simulink model "EKF"  (R2021b)
settings: Solver=ode4  StartTime=0.0  StopTime=200  FixedStep=0.02  RelTol=1e-3
libraries: commchan3 x2
(part 2 of 4)

== matlab function EKF/MATLAB Function3 ==
  data: y input; xhat output; u input; Pcov output; xhat input
function [xhat, Pcov]= fcn(y, u, xhat)
    Ts = 0.02;
    Qk = eye(5);
    Qk(1,1) = 1e-8;
    Qk(2,2) = 1e-8;
    Qk(3,3) = 1e-8;
    Qk(4,4) = 1e-5;
    Qk(5,5) = 1e-2;
    Rk = 1e-6;
    C = [0, 1, 0, 0, 0];
    n = 5; % dimension of state space
    lambda=(alpha)^2+(n+k)-n;
    alpha=1e-3;
    beta = 2;
    k=0;

   
    W_0m=lambda/(n+lambda);
    W_0c=W_mo+(1-(alpha)^2+beta);

%     for i = 1:2*n
        W_0m1 = 1/(2*(n+lambda));
%     end
    
   
    persistent xhat_p mhat_p Pcov_p xhata_p phata_p;

    % initialization
    if isempty(xhat_p)
        xhat_p = [0;0;0;1/2;4];
        Pcov_p = (xhat_p - mhat_p)* (xhat_p - mhat_p)';
    end

    W_0m=lambda/(n+lambda);
    x_sigma0 = xhat_p;
    x_sigma1 = zeros(5,1);
    x_sigma2 = zeros(5,1);
%     x_sigma = zeros(10,1);

    for i=1:n
        x_sigma1(i) = xhat_p+sqrt((n+lambda)*Pcov_p(i));
    end

    for i=n+1:2*n
        x_sigma2(i) = xhat_p-sqrt((n+lambda)*Pcov_p(i));
    end
    

%    xkm = Fd(x_sigma, u, Ts);
    x_prior=zeros(5,1);
    x_prior1=zeros(5,1);
    x_prior2=zeros(5,1);
    x_prior3=zeros(5,1);
    P_prior=zeros(5,5);
    P_prior1=zeros(5,5);
    P_prior2=zeros(5,5);
    P_prior3=zeros(5,5);
    y_prior=zeros(5,1);

    for i = 1:(2*n+1)
        if i == 1
            x_prior1 = x_prior + W_0m * x_sigma0;
        elseif i > 1 && i <= n
            x_prior2(i) =  x_prior2(i) + W_0m1 *x_sigma1(i);
        elseif i > n && i <= (2*n+1)
             x_prior3(i) =  x_prior3(i) + W_0m1 *x_sigma2(i);
        end
    end

    x_prior = x_prior1 + x_prior2 + x_prior3;

   for i = 1:(2*n+1)
        if i == 1
            P_prior1 = P_prior1 + W_0c * [x_sigma0 - x_prior] * [x_sigma0 - x_prior]';
        elseif i > 1 && i <= n
            P_prior2(i) = P_prior2(i) + W_0m1   * [x_sigma1(i) - x_prior] * [x_sigma1(i) - x_prior]';
        elseif i > n && i <= (2*n+1)
            P_prior3(i) = P_prior3(i) + W_0m1   * [x_sigma3(i) - x_prior] * [x_sigma3(i) - x_prior]';
        end
   end

   P_prior = P_prior1 + P_prior2 + P_prior3;

 y_sigma0 = y;
    y_sigma1 = zeros(5,1);
    y_sigma2 = zeros(5,1);


    for i=1:n
        y_sigma1(i) = y+sqrt((n+lambda)*Pcov_p(i));
    end

    for i=n+1:2*n
        y_sigma2(i) = y-sqrt((n+lambda)*Pcov_p(i));
    end

     y_prior=zeros(5,1);
    y_prior1=zeros(5,1);
    y_prior2=zeros(5,1);
    y_prior3=zeros(5,1);
for i = 1:(2*n+1)
        if i == 1
            y_prior1 = y_prior + W_0m1 * y_sigma0;
        elseif i > 1 && i <= n
            y_prior2(i) =  y_prior2(i) + W_0m1 *y_sigma1(i);
        elseif i > n && i <= (2*n+1)
             y_prior3(i) =  y_prior3(i) + W_0m1 *y_sigma2(i);
        end
    end
end
    y_prior = y_prior1 + y_prior2 + y_prior3;

    %measurement update
    Pyy=zeros(5,5);
    Pxy=zeros(5,5);

   
   for i = 1:(2*n+1)
        if i == 1
            P_prior1 = P_prior1 + W_0c * [y_sigma0 - y_prior] * [x_sigma0 - x_prior]';
        elseif i > 1 && i <= n
            P_prior2(i) = P_prior2(i) + W_0m1   * [x_sigma1(i) - x_prior] * [x_sigma1(i) - x_prior]';
        elseif i > n && i <= (2*n+1)
            P_prior3(i) = P_prior3(i) + W_0m1   * [x_sigma3(i) - x_prior] * [x_sigma3(i) - x_prior]';
        end
   end

   P_prior = P_prior1 + P_prior2 + P_prior3

%     
%     Fk = J_wrtX(xhat_p, u, Ts);
%     Pkm = Fk*Pcov_p*Fk' + Qk;
%     
%     y_err = y - C*xkm;
%     Sk = C*Pkm*C' + Rk;
%     Kk = Pkm * C'*inv(Sk);
%     xhat = xkm + Kk*y_err;
%     Pcov_final = (eye(5) - Kk*C)*Pkm;
%     
%     Pcov = reshape(Pcov_final, [25, 1]);
%     
%     xhat_p = xhat;
%     Pcov_p = Pcov_final;
% 
%     function X1 = Fd(x, u, Ts)
%         x1 = x(1);
%         x2 = x(2);
%         x3 = x(3);
%         M = x(4);
%         D = x(5);
%         X1 = [x1 + (Ts*(6*x2 + Ts*x3 + Ts*(x3 - (Ts*(5*M*u + (x2 + (Ts*x3)/2)*(100*M + 5*D*M) + 10*M*(x1 + (Ts*x2)/2) + (x3 - (Ts*(5*M*u + 10*M*x1 + x3*(D*M + 5) + x2*(100*M + 5*D*M)))/2)*(D*M + 5)))/2) + Ts*(x3 - (Ts*(5*M*u + 10*M*x1 + x3*(D*M + 5) + x2*(100*M + 5*D*M)))/2)))/6;
%              x2 - (Ts*(Ts*(5*M*u + (x2 + (Ts*x3)/2)*(100*M + 5*D*M) + 10*M*(x1 + (Ts*x2)/2) + (x3 - (Ts*(5*M*u + 10*M*x1 + x3*(D*M + 5) + x2*(100*M + 5*D*M)))/2)*(D*M + 5)) - 6*x3 + Ts*((x2 + (Ts*(x3 - (Ts*(5*M*u + 10*M*x1 + x3*(D*M + 5) + x2*(100*M + 5*D*M)))/2))/2)*(100*M + 5*D*M) + 5*M*u + 10*M*(x1 + (Ts*(x2 + (Ts*x3)/2))/2) + (D*M + 5)*(x3 - (Ts*(5*M*u + (x2 + (Ts*x3)/2)*(100*M + 5*D*M) + 10*M*(x1 + (Ts*x2)/2) + (x3 - (Ts*(5*M*u + 10*M*x1 + x3*(D*M + 5) + x2*(100*M + 5*D*M)))/2)*(D*M + 5)))/2)) + Ts*(5*M*u + 10*M*x1 + x3*(D*M + 5) + x2*(100*M + 5*D*M))))/6;
%              x3 - (Ts*(2*(x2 + (Ts*(x3 - (Ts*(5*M*u + 10*M*x1 + x3*(D*M + 5) + x2*(100*M + 5*D*M)))/2))/2)*(100*M + 5*D*M) + 30*M*u + 10*M*x1 + x3*(D*M + 5) + 20*M*(x1 + (Ts*(x2 + (Ts*x3)/2))/2) + 2*(x2 + (Ts*x3)/2)*(100*M + 5*D*M) + 2*(D*M + 5)*(x3 - (Ts*(5*M*u + (x2 + (Ts*x3)/2)*(100*M + 5*D*M) + 10*M*(x1 + (Ts*x2)/2) + (x3 - (Ts*(5*M*u + 10*M*x1 + x3*(D*M + 5) + x2*(100*M + 5*D*M)))/2)*(D*M + 5)))/2) + 20*M*(x1 + (Ts*x2)/2) + (x3 - Ts*((x2 + (Ts*(x3 - (Ts*(5*M*u + 10*M*x1 + x3*(D*M + 5) + x2*(100*M + 5*D*M)))/2))/2)*(100*M + 5*D*M) + 5*M*u + 10*M*(x1 + (Ts*(x2 + (Ts*x3)/2))/2) + (D*M + 5)*(x3 - (Ts*(5*M*u + (x2 + (Ts*x3)/2)*(100*M + 5*D*M) + 10*M*(x1 + (Ts*x2)/2) + (x3 - (Ts*(5*M*u + 10*M*x1 + x3*(D*M + 5) + x2*(100*M + 5*D*M)))/2)*(D*M + 5)))/2)))*(D*M + 5) + x2*(100*M + 5*D*M) + 2*(x3 - (Ts*(5*M*u + 10*M*x1 + x3*(D*M + 5) + x2*(100*M + 5*D*M)))/2)*(D*M + 5) + (x2 + Ts*(x3 - (Ts*(5*M*u + (x2 + (Ts*x3)/2)*(100*M + 5*D*M) + 10*M*(x1 + (Ts*x2)/2) + (x3 - (Ts*(5*M*u + 10*M*x1 + x3*(D*M + 5) + x2*(100*M + 5*D*M)))/2)*(D*M + 5)))/2))*(100*M + 5*D*M) + 10*M*(x1 + Ts*(x2 + (Ts*(x3 - (Ts*(5*M*u + 10*M*x1 + x3*(D*M + 5) + x2*(100*M + 5*D*M)))/2))/2))))/6;
%              M;
%              D];
%     end
% 
%     function Ad = J_wrtX(x, u, Ts)
%         x1 = x(1);
%         x2 = x(2);
%         x3 = x(3);
%         M = x(4);
%         D = x(5);
%         Ad = [1 - (Ts*(5*M*Ts^2 + (Ts^2*(10*M - 5*M*Ts*(D*M + 5)))/2))/6,-(Ts*((Ts^2*(100*M + 5*D*M))/2 + (Ts^2*(100*M + 5*M*Ts + 5*D*M - (Ts*(D*M + 5)*(100*M + 5*D*M))/2))/2 - 6))/6, (Ts*(Ts - Ts*((Ts*(D*M + 5))/2 - 1) + Ts*((Ts*((D*M + 5)*((Ts*(D*M + 5))/2 - 1) - (Ts*(100*M + 5*D*M))/2))/2 + 1)))/6, -(Ts*((Ts^2*(5*u + 10*x1 + D*x3 + x2*(5*D + 100)))/2 + (Ts^2*(5*u + 10*x1 + 5*Ts*x2 + (5*D + 100)*(x2 + (Ts*x3)/2) + D*(x3 - (Ts*(5*M*u + 10*M*x1 + x3*(D*M + 5) + x2*(100*M + 5*D*M)))/2) - (Ts*(D*M + 5)*(5*u + 10*x1 + D*x3 + x2*(5*D + 100)))/2))/2))/6,-(Ts*((Ts^2*(5*M*(x2 + (Ts*x3)/2) + M*(x3 - (Ts*(5*M*u + 10*M*x1 + x3*(D*M + 5) + x2*(100*M + 5*D*M)))/2) - (Ts*(D*M + 5)*(5*M*x2 + M*x3))/2))/2 + (Ts^2*(5*M*x2 + M*x3))/2))/6;
%             -(Ts*(10*M*Ts + Ts*(10*M - 5*M*Ts*(D*M + 5)) - Ts*((5*M*Ts^2*(100*M + 5*D*M))/2 - 10*M + (Ts*(D*M + 5)*(10*M - 5*M*Ts*(D*M + 5)))/2)))/6, 1 - (Ts*(Ts*(100*M + 5*D*M) + Ts*(100*M + 5*M*Ts + 5*D*M - (Ts*(D*M + 5)*(100*M + 5*D*M))/2) - Ts*(((Ts^2*(100*M + 5*D*M))/4 - 1)*(100*M + 5*D*M) - 5*M*Ts + (Ts*(D*M + 5)*(100*M + 5*M*Ts + 5*D*M - (Ts*(D*M + 5)*(100*M + 5*D*M))/2))/2)))/6,-(Ts*(Ts*(D*M + 5) + Ts*((5*M*Ts^2)/2 + ((Ts*((D*M + 5)*((Ts*(D*M + 5))/2 - 1) - (Ts*(100*M + 5*D*M))/2))/2 + 1)*(D*M + 5) - (Ts*((Ts*(D*M + 5))/2 - 1)*(100*M + 5*D*M))/2) - Ts*((D*M + 5)*((Ts*(D*M + 5))/2 - 1) - (Ts*(100*M + 5*D*M))/2) - 6))/6, -(Ts*(Ts*(5*u + 10*x1 + 5*Ts*x2 + (5*D + 100)*(x2 + (Ts*x3)/2) + D*(x3 - (Ts*(5*M*u + 10*M*x1 + x3*(D*M + 5) + x2*(100*M + 5*D*M)))/2) - (Ts*(D*M + 5)*(5*u + 10*x1 + D*x3 + x2*(5*D + 100)))/2) + Ts*(5*u + 10*x1 + (5*D + 100)*(x2 + (Ts*(x3 - (Ts*(5*M*u + 10*M*x1 + x3*(D*M + 5) + x2*(100*M + 5*D*M)))/2))/2) + D*(x3 - (Ts*(5*M*u + (x2 + (Ts*x3)/2)*(100*M + 5*D*M) + 10*M*(x1 + (Ts*x2)/2) + (x3 - (Ts*(5*M*u + 10*M*x1 + x3*(D*M + 5) + x2*(100*M + 5*D*M)))/2)*(D*M + 5)))/2) + 5*Ts*(x2 + (Ts*x3)/2) - (Ts^2*(100*M + 5*D*M)*(5*u + 10*x1 + D*x3 + x2*(5*D + 100)))/4 - (Ts*(D*M + 5)*(5*u + 10*x1 + 5*Ts*x2 + (5*D + 100)*(x2 + (Ts*x3)/2) + D*(x3 - (Ts*(5*M*u + 10*M*x1 + x3*(D*M + 5) + x2*(100*M + 5*D*M)))/2) - (Ts*(D*M + 5)*(5*u + 10*x1 + D*x3 + x2*(5*D + 100)))/2))/2) + Ts*(5*u + 10*x1 + D*x3 + x2*(5*D + 100))))/6,-(Ts*(Ts*(5*M*(x2 + (Ts*x3)/2) + M*(x3 - (Ts*(5*M*u + 10*M*x1 + x3*(D*M + 5) + x2*(100*M + 5*D*M)))/2) - (Ts*(D*M + 5)*(5*M*x2 + M*x3))/2) + Ts*(5*M*x2 + M*x3) + Ts*(5*M*(x2 + (Ts*(x3 - (Ts*(5*M*u + 10*M*x1 + x3*(D*M + 5) + x2*(100*M + 5*D*M)))/2))/2) + M*(x3 - (Ts*(5*M*u + (x2 + (Ts*x3)/2)*(100*M + 5*D*M) + 10*M*(x1 + (Ts*x2)/2) + (x3 - (Ts*(5*M*u + 10*M*x1 + x3*(D*M + 5) + x2*(100*M + 5*D*M)))/2)*(D*M + 5)))/2) - (Ts*(D*M + 5)*(5*M*(x2 + (Ts*x3)/2) + M*(x3 - (Ts*(5*M*u + 10*M*x1 + x3*(D*M + 5) + x2*(100*M + 5*D*M)))/2) - (Ts*(D*M + 5)*(5*M*x2 + M*x3))/2))/2 - (Ts^2*(5*M*x2 + M*x3)*(100*M + 5*D*M))/4)))/6;
%             (Ts*(10*M*((5*M*Ts^3)/2 - 1) - 50*M + 10*M*Ts*(D*M + 5) + 5*M*Ts^2*(100*M + 5*D*M) + Ts*(D*M + 5)*(10*M - 5*M*Ts*(D*M + 5)) + (Ts^2*(10*M - 5*M*Ts*(D*M + 5))*(100*M + 5*D*M))/2 - Ts*(D*M + 5)*((5*M*Ts^2*(100*M + 5*D*M))/2 - 10*M + (Ts*(D*M + 5)*(10*M - 5*M*Ts*(D*M + 5)))/2)))/6, (Ts*(2*((Ts^2*(100*M + 5*D*M))/4 - 1)*(100*M + 5*D*M) - 20*M*Ts - 300*M + ((Ts^2*(100*M + 5*M*Ts + 5*D*M - (Ts*(D*M + 5)*(100*M + 5*D*M))/2))/2 - 1)*(100*M + 5*D*M) - 15*D*M + Ts*(D*M + 5)*(100*M + 5*D*M) + Ts*(D*M + 5)*(100*M + 5*M*Ts + 5*D*M - (Ts*(D*M + 5)*(100*M + 5*D*M))/2) - Ts*(D*M + 5)*(((Ts^2*(100*M + 5*D*M))/4 - 1)*(100*M + 5*D*M) - 5*M*Ts + (Ts*(D*M + 5)*(100*M + 5*M*Ts + 5*D*M - (Ts*(D*M + 5)*(100*M + 5*D*M))/2))/2) + 10*M*Ts*((Ts^2*(100*M + 5*D*M))/4 - 1)))/6, 1 - (Ts*(5*M*Ts^2 - 2*(D*M + 5)*((Ts*(D*M + 5))/2 - 1) - (D*M + 5)*(Ts*((5*M*Ts^2)/2 + ((Ts*((D*M + 5)*((Ts*(D*M + 5))/2 - 1) - (Ts*(100*M + 5*D*M))/2))/2 + 1)*(D*M + 5) - (Ts*((Ts*(D*M + 5))/2 - 1)*(100*M + 5*D*M))/2) - 1) + Ts*(100*M + 5*D*M) + 2*((Ts*((D*M + 5)*((Ts*(D*M + 5))/2 - 1) - (Ts*(100*M + 5*D*M))/2))/2 + 1)*(D*M + 5) + D*M - Ts*((Ts*(D*M + 5))/2 - 1)*(100*M + 5*D*M) - 5*M*Ts^2*((Ts*(D*M + 5))/2 - 1) + Ts*((Ts*((D*M + 5)*((Ts*(D*M + 5))/2 - 1) - (Ts*(100*M + 5*D*M))/2))/2 + 1)*(100*M + 5*D*M) + 5))/6, -(Ts*(30*u + 60*x1 + 2*(5*D + 100)*(x2 + (Ts*(x3 - (Ts*(5*M*u + 10*M*x1 + x3*(D*M + 5) + x2*(100*M + 5*D*M)))/2))/2) + D*x3 + 10*Ts*x2 + 2*(5*D + 100)*(x2 + (Ts*x3)/2) + 10*Ts*(x2 + (Ts*(x3 - (Ts*(5*M*u + 10*M*x1 + x3*(D*M + 5) + x2*(100*M + 5*D*M)))/2))/2) + 2*D*(x3 - (Ts*(5*M*u + (x2 + (Ts*x3)/2)*(100*M + 5*D*M) + 10*M*(x1 + (Ts*x2)/2) + (x3 - (Ts*(5*M*u + 10*M*x1 + x3*(D*M + 5) + x2*(100*M + 5*D*M)))/2)*(D*M + 5)))/2) + D*(x3 - Ts*((x2 + (Ts*(x3 - (Ts*(5*M*u + 10*M*x1 + x3*(D*M + 5) + x2*(100*M + 5*D*M)))/2))/2)*(100*M + 5*D*M) + 5*M*u + 10*M*(x1 + (Ts*(x2 + (Ts*x3)/2))/2) + (D*M + 5)*(x3 - (Ts*(5*M*u + (x2 + (Ts*x3)/2)*(100*M + 5*D*M) + 10*M*(x1 + (Ts*x2)/2) + (x3 - (Ts*(5*M*u + 10*M*x1 + x3*(D*M + 5) + x2*(100*M + 5*D*M)))/2)*(D*M + 5)))/2))) + 10*Ts*(x2 + (Ts*x3)/2) + 2*D*(x3 - (Ts*(5*M*u + 10*M*x1 + x3*(D*M + 5) + x2*(100*M + 5*D*M)))/2) + x2*(5*D + 100) + (5*D + 100)*(x2 + Ts*(x3 - (Ts*(5*M*u + (x2 + (Ts*x3)/2)*(100*M + 5*D*M) + 10*M*(x1 + (Ts*x2)/2) + (x3 - (Ts*(5*M*u + 10*M*x1 + x3*(D*M + 5) + x2*(100*M + 5*D*M)))/2)*(D*M + 5)))/2)) - Ts*(D*M + 5)*(5*u + 10*x1 + (5*D + 100)*(x2 + (Ts*(x3 - (Ts*(5*M*u + 10*M*x1 + x3*(D*M + 5) + x2*(100*M + 5*D*M)))/2))/2) + D*(x3 - (Ts*(5*M*u + (x2 + (Ts*x3)/2)*(100*M + 5*D*M) + 10*M*(x1 + (Ts*x2)/2) + (x3 - (Ts*(5*M*u + 10*M*x1 + x3*(D*M + 5) + x2*(100*M + 5*D*M)))/2)*(D*M + 5)))/2) + 5*Ts*(x2 + (Ts*x3)/2) - (Ts^2*(100*M + 5*D*M)*(5*u + 10*x1 + D*x3 + x2*(5*D + 100)))/4 - (Ts*(D*M + 5)*(5*u + 10*x1 + 5*Ts*x2 + (5*D + 100)*(x2 + (Ts*x3)/2) + D*(x3 - (Ts*(5*M*u + 10*M*x1 + x3*(D*M + 5) + x2*(100*M + 5*D*M)))/2) - (Ts*(D*M + 5)*(5*u + 10*x1 + D*x3 + x2*(5*D + 100)))/2))/2) - Ts*(D*M + 5)*(5*u + 10*x1 + D*x3 + x2*(5*D + 100)) - (Ts^2*(100*M + 5*D*M)*(5*u + 10*x1 + D*x3 + x2*(5*D + 100)))/2 - (5*M*Ts^3*(5*u + 10*x1 + D*x3 + x2*(5*D + 100)))/2 - Ts*(D*M + 5)*(5*u + 10*x1 + 5*Ts*x2 + (5*D + 100)*(x2 + (Ts*x3)/2) + D*(x3 - (Ts*(5*M*u + 10*M*x1 + x3*(D*M + 5) + x2*(100*M + 5*D*M)))/2) - (Ts*(D*M + 5)*(5*u + 10*x1 + D*x3 + x2*(5*D + 100)))/2) - (Ts^2*(100*M + 5*D*M)*(5*u + 10*x1 + 5*Ts*x2 + (5*D + 100)*(x2 + (Ts*x3)/2) + D*(x3 - (Ts*(5*M*u + 10*M*x1 + x3*(D*M + 5) + x2*(100*M + 5*D*M)))/2) - (Ts*(D*M + 5)*(5*u + 10*x1 + D*x3 + x2*(5*D + 100)))/2))/2))/6, -(Ts*(5*M*x2 + M*x3 + 5*M*(x2 + Ts*(x3 - (Ts*(5*M*u + (x2 + (Ts*x3)/2)*(100*M + 5*D*M) + 10*M*(x1 + (Ts*x2)/2) + (x3 - (Ts*(5*M*u + 10*M*x1 + x3*(D*M + 5) + x2*(100*M + 5*D*M)))/2)*(D*M + 5)))/2)) + 10*M*(x2 + (Ts*(x3 - (Ts*(5*M*u + 10*M*x1 + x3*(D*M + 5) + x2*(100*M + 5*D*M)))/2))/2) + 2*M*(x3 - (Ts*(5*M*u + (x2 + (Ts*x3)/2)*(100*M + 5*D*M) + 10*M*(x1 + (Ts*x2)/2) + (x3 - (Ts*(5*M*u + 10*M*x1 + x3*(D*M + 5) + x2*(100*M + 5*D*M)))/2)*(D*M + 5)))/2) + M*(x3 - Ts*((x2 + (Ts*(x3 - (Ts*(5*M*u + 10*M*x1 + x3*(D*M + 5) + x2*(100*M + 5*D*M)))/2))/2)*(100*M + 5*D*M) + 5*M*u + 10*M*(x1 + (Ts*(x2 + (Ts*x3)/2))/2) + (D*M + 5)*(x3 - (Ts*(5*M*u + (x2 + (Ts*x3)/2)*(100*M + 5*D*M) + 10*M*(x1 + (Ts*x2)/2) + (x3 - (Ts*(5*M*u + 10*M*x1 + x3*(D*M + 5) + x2*(100*M + 5*D*M)))/2)*(D*M + 5)))/2))) + 10*M*(x2 + (Ts*x3)/2) + 2*M*(x3 - (Ts*(5*M*u + 10*M*x1 + x3*(D*M + 5) + x2*(100*M + 5*D*M)))/2) - (5*M*Ts^3*(5*M*x2 + M*x3))/2 - Ts*(D*M + 5)*(5*M*(x2 + (Ts*x3)/2) + M*(x3 - (Ts*(5*M*u + 10*M*x1 + x3*(D*M + 5) + x2*(100*M + 5*D*M)))/2) - (Ts*(D*M + 5)*(5*M*x2 + M*x3))/2) - (Ts^2*(100*M + 5*D*M)*(5*M*(x2 + (Ts*x3)/2) + M*(x3 - (Ts*(5*M*u + 10*M*x1 + x3*(D*M + 5) + x2*(100*M + 5*D*M)))/2) - (Ts*(D*M + 5)*(5*M*x2 + M*x3))/2))/2 - Ts*(D*M + 5)*(5*M*x2 + M*x3) - (Ts^2*(5*M*x2 + M*x3)*(100*M + 5*D*M))/2 - Ts*(D*M + 5)*(5*M*(x2 + (Ts*(x3 - (Ts*(5*M*u + 10*M*x1 + x3*(D*M + 5) + x2*(100*M + 5*D*M)))/2))/2) + M*(x3 - (Ts*(5*M*u + (x2 + (Ts*x3)/2)*(100*M + 5*D*M) + 10*M*(x1 + (Ts*x2)/2) + (x3 - (Ts*(5*M*u + 10*M*x1 + x3*(D*M + 5) + x2*(100*M + 5*D*M)))/2)*(D*M + 5)))/2) - (Ts*(D*M + 5)*(5*M*(x2 + (Ts*x3)/2) + M*(x3 - (Ts*(5*M*u + 10*M*x1 + x3*(D*M + 5) + x2*(100*M + 5*D*M)))/2) - (Ts*(D*M + 5)*(5*M*x2 + M*x3))/2))/2 - (Ts^2*(5*M*x2 + M*x3)*(100*M + 5*D*M))/4)))/6;
%             0,0, 0, 1,0;
%             0,0, 0, 0,1];
%     end
end
